simulink model "running_avg_TB"  (R2024a)
settings: Solver=VariableStepAuto  StartTime=0.0  StopTime=2000  RelTol=1e-3
libraries: dspsrcs4 x1
settings Model: Creator=kschutz  LastModifiedBy=kschutz

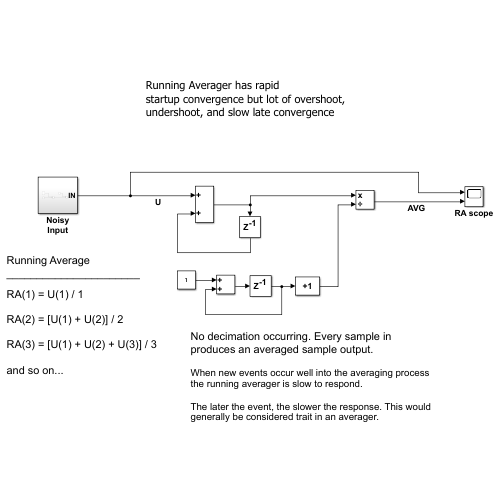
[thumbnail: Simulink's stored preview of the top-level diagram]
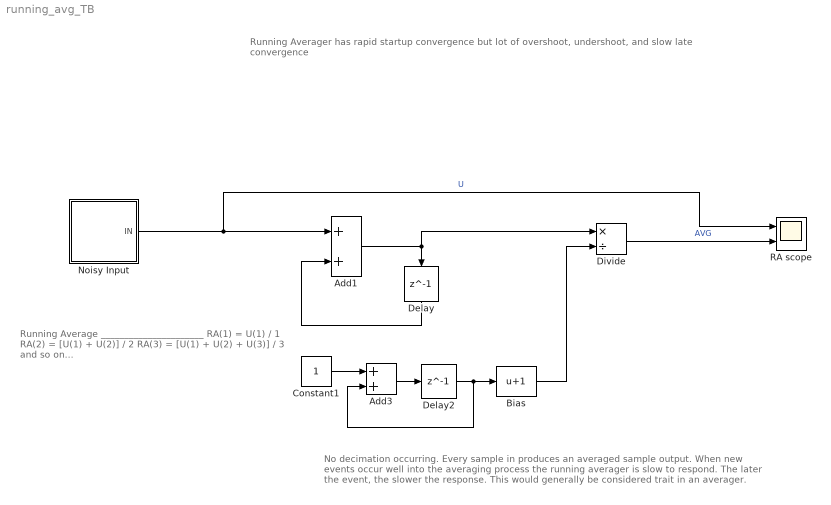
== system running_avg_TB ==
  note: No decimation occurring. Every sample in produces an averaged sample output.
      |
      | When new events occur well into the averaging process the running averager is slow to respond.
      |
      | The later the event, the slower the response. This would generally be considered trait in an averager.
  note: Running Averager has rapid
      | startup convergence but lot of overshoot, undershoot, and slow late convergence
  note: Running Average
      | ______________________
      |
      | RA(1) = U(1) / 1
      |
      | RA(2) = [U(1) + U(2)] / 2
      |
      | RA(3) = [U(1) + U(2) + U(3)] / 3
      |
      | and so on...
  Add1 : Sum
  Add3 : Sum
  Bias : Bias  Bias=1  SaturateOnIntegerOverflow=off
  Constant1 : Constant
  Delay : Delay  DelayLength=1
  Delay2 : Delay  DelayLength=1  InitialCondition=0
  Divide : Product  Inputs=*/
  Noisy Input : Subsystem
  RA scope : Scope  NumInputPorts=2
  wires:
  Bias/1 -> Divide/2
  Constant1/1 -> Add3/1
  Add3/1 -> Delay2/1
  Delay2/1 -> Add3/2, Bias/1
  Divide/1 -> RA scope/2  "AVG"
  Noisy Input/1(IN) -> RA scope/1, Add1/1  "U"
  Delay/1 -> Add1/2
  Add1/1 -> Divide/1, Delay/1

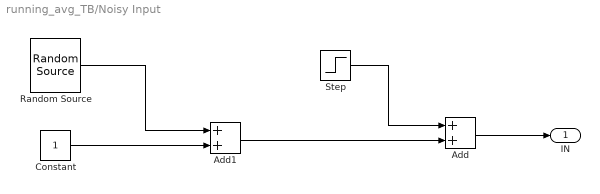
== system running_avg_TB/Noisy Input ==
  Add : Sum
  Add1 : Sum
  Constant : Constant  SampleTime=1
  Random Source : dspsrcs4/Random Source  SrcType=Gaussian  MinVal=0  MaxVal=1  MeanVal=0  VarVal=.2  RepMode=Specify seed  rawSeed=123  IsInherit=off  SampTime=1  SampFrame=1  OutComplex=Real  DataType=double  SimulateUsing=Interpreted execution
  Step : Step  Time=500  SampleTime=0
  IN : Outport  VectorParamsAs1DForOutWhenUnconnected=off
  wires:
  Constant/1 -> Add1/2
  Random Source/1 -> Add1/1
  Add/1 -> IN/1
  Add1/1 -> Add/2
  Step/1 -> Add/1
